simulink model "component_model_with_requirements"  (R2019b)
settings: Solver=VariableStepAuto  StartTime=0.0  StopTime=inf  RelTol=1e-3
settings Model: Creator=anton  LastModifiedBy=scarcia
settings SFSimCC: CustomCodeUndefinedFunction=UseInterfaceOnly

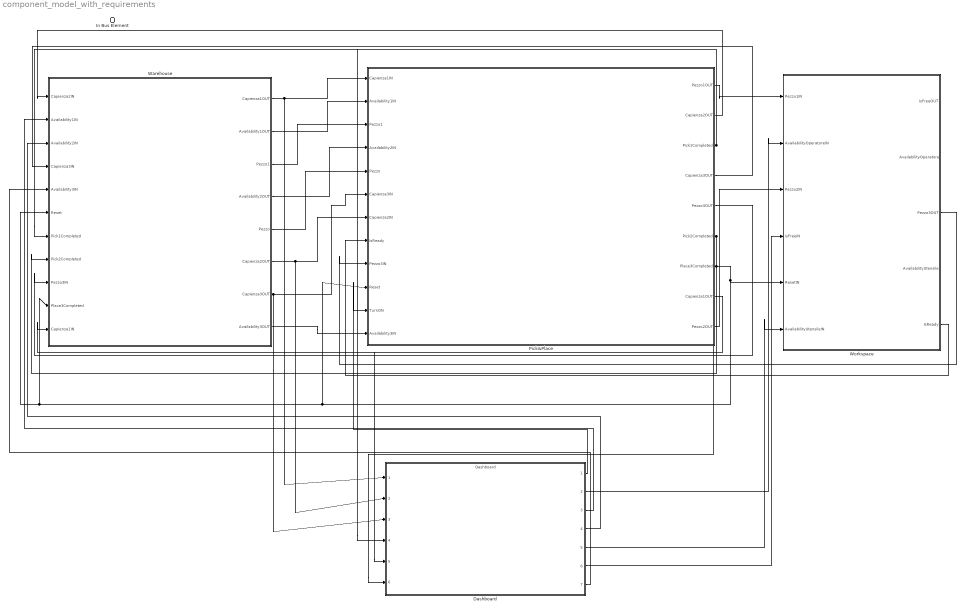
== system component_model_with_requirements ==
  In Bus Element : Inport  PortName=InBus
  Dashboard : ModelReference  ModelNameDialog=Dashboard  SimulationMode=Normal  ModelReferenceVersion=1.7
      settings: PortSchema="{\"entries\":[{\"content\":{\"headerSize\":38,\"margin\":15,\"minimumSpacing\":25,\"sides\":[{\"content\":{\"connectorIds\":[\"In1\",\"In2\",\"In3\",\"In4\",\"In5\",\"In6\"]},\"type\":\"ConnectorPlacement.EquallySpacedRectSide\",\"uuid\":\"84c4e9a6-c7e3-4ff5-8779-8f22ff7ec920\"},{\"content\":{\"connectorIds\":[\"Out1\",\"Out2\",\"Out3\",\"Out4\",\"Out5\",\"Out6\",\"Out7\"],\"side\":\"RIGHT\"},\"type\":\"ConnectorPlacement.EquallySpacedRectSide\",\"uuid\":\"3a8574bf-2f52-453d-9cac-f8720b3c2634\"},{\"content\":{\"connectorIds\":[],\"side\":\"TOP\"},\"type\":\"ConnectorPlacement.EquallySpacedRectSide\",\"uuid\":\"c01d23e2-01e7-488d-9b06-220ab7823b69\"}]},\"type\":\"ConnectorPlacement.EquallySpacedConnector\",\"uuid\":\"4b97af20-a068-43b9-acb3-094aa2dc4c50\"}],\"packageUris\":[\"http:\\/\\/schema.mathworks.com\\/mf0\\/Connector\\/19700101\"],\"version\":\"1.0\"}"
  Pick&Place : Subsystem
      settings: PortSchema="{\"entries\":[{\"content\":{\"headerSize\":26,\"margin\":15,\"minimumSpacing\":25,\"sides\":[{\"content\":{\"connectorIds\":[\"In1\",\"In2\",\"In3\",\"In4\",\"In5\",\"In6\",\"In7\",\"In8\",\"In9\",\"In10\",\"In11\",\"In12\"]},\"type\":\"ConnectorPlacement.EquallySpacedRectSide\",\"uuid\":\"cd5611c0-8a30-4803-bae5-8792d5ed3138\"},{\"content\":{\"connectorIds\":[\"Out1\",\"Out2\",\"Out3\",\"Out4\",\"Out5\",\"Out6\",\"Out7\",\"Out8\",\"Out9\"],\"side\":\"RIGHT\"},\"type\":\"ConnectorPlacement.EquallySpacedRectSide\",\"uuid\":\"19615e04-708c-4dc8-9217-130af3d4c815\"},{\"content\":{\"connectorIds\":[],\"side\":\"TOP\"},\"type\":\"ConnectorPlacement.EquallySpacedRectSide\",\"uuid\":\"bde4fae3-4c2b-4ff8-8efa-5dc73cdd4226\"},{\"content\":{\"connectorIds\":[],\"side\":\"BOTTOM\"},\"type\":\"ConnectorPlacement.EquallySpacedRectSide\",\"uuid\":\"49cfc24f-8487-4a02-9b01-8a859a4a9c32\"}]},\"type\":\"ConnectorPlacement.EquallySpacedConnector\",\"uuid\":\"74f0ebde-c382-4fb1-af99-ecf6372bc12c\"}],\"packageUris\":[\"http:\\/\\/schema.mathworks.com\\/mf0\\/Connector\\/19700101\"],\"version\":\"1.0\"}"
  Warehouse : Subsystem
      settings: PortSchema="{\"entries\":[{\"content\":{\"headerSize\":26,\"margin\":15,\"minimumSpacing\":25,\"sides\":[{\"content\":{\"connectorIds\":[\"In1\",\"In2\",\"In3\",\"In4\",\"In5\",\"In6\",\"In7\",\"In8\",\"In9\",\"In10\",\"In11\"]},\"type\":\"ConnectorPlacement.EquallySpacedRectSide\",\"uuid\":\"cd5611c0-8a30-4803-bae5-8792d5ed3138\"},{\"content\":{\"connectorIds\":[\"Out1\",\"Out2\",\"Out3\",\"Out4\",\"Out5\",\"Out6\",\"Out7\",\"Out8\"],\"side\":\"RIGHT\"},\"type\":\"ConnectorPlacement.EquallySpacedRectSide\",\"uuid\":\"19615e04-708c-4dc8-9217-130af3d4c815\"},{\"content\":{\"connectorIds\":[],\"side\":\"TOP\"},\"type\":\"ConnectorPlacement.EquallySpacedRectSide\",\"uuid\":\"bde4fae3-4c2b-4ff8-8efa-5dc73cdd4226\"}]},\"type\":\"ConnectorPlacement.EquallySpacedConnector\",\"uuid\":\"74f0ebde-c382-4fb1-af99-ecf6372bc12c\"}],\"packageUris\":[\"http:\\/\\/schema.mathworks.com\\/mf0\\/Connector\\/19700101\"],\"version\":\"1.0\"}"
  Workspace : Subsystem
      settings: PortSchema="{\"entries\":[{\"content\":{\"headerSize\":26,\"margin\":15,\"minimumSpacing\":25,\"sides\":[{\"content\":{\"connectorIds\":[\"In1\",\"In2\",\"In3\",\"In4\",\"In5\",\"In6\"]},\"type\":\"ConnectorPlacement.EquallySpacedRectSide\",\"uuid\":\"cd5611c0-8a30-4803-bae5-8792d5ed3138\"},{\"content\":{\"connectorIds\":[\"Out1\",\"Out2\",\"Out3\",\"Out4\",\"Out5\"],\"side\":\"RIGHT\"},\"type\":\"ConnectorPlacement.EquallySpacedRectSide\",\"uuid\":\"19615e04-708c-4dc8-9217-130af3d4c815\"},{\"content\":{\"connectorIds\":[],\"side\":\"TOP\"},\"type\":\"ConnectorPlacement.EquallySpacedRectSide\",\"uuid\":\"bde4fae3-4c2b-4ff8-8efa-5dc73cdd4226\"}]},\"type\":\"ConnectorPlacement.EquallySpacedConnector\",\"uuid\":\"74f0ebde-c382-4fb1-af99-ecf6372bc12c\"}],\"packageUris\":[\"http:\\/\\/schema.mathworks.com\\/mf0\\/Connector\\/19700101\"],\"version\":\"1.0\"}"
  wires:
  Pick&Place/8(Capienza1OUT) -> Warehouse/11(Capienza1IN)
  Pick&Place/2(Capienza2OUT) -> Warehouse/1(Capienza2IN)
  Pick&Place/4(Capienza3OUT) -> Warehouse/4(Capienza3IN)
  Warehouse/1(Capienza1OUT) -> Pick&Place/1(Capienza1IN), Dashboard/1
  Warehouse/6(Capienza2OUT) -> Pick&Place/7(Capienza2IN), Dashboard/2
  Warehouse/3(Pezzo1) -> Pick&Place/3(Pezzo1)
  Warehouse/5(Pezzo) -> Pick&Place/5(Pezzo)
  Warehouse/2(Availability1OUT) -> Pick&Place/2(Availability1IN)
  Warehouse/4(Availability2OUT) -> Pick&Place/4(Availability2IN)
  Warehouse/7(Capienza3OUT) -> Pick&Place/6(Capienza3IN), Dashboard/3
  Pick&Place/1(Pezzo1OUT) -> Workspace/1(Pezzo1IN)
  Pick&Place/9(Pezzo2OUT) -> Workspace/3(Pezzo2IN)
  Workspace/5(IsReady) -> Pick&Place/8(IsReady)
  Workspace/3(Pezzo3OUT) -> Pick&Place/9(Pezzo3IN)
  Pick&Place/5(Pezzo3OUT) -> Warehouse/9(Pezzo3IN)
  Warehouse/8(Availability3OUT) -> Pick&Place/12(Availability3IN)
  Pick&Place/6(Pick2Completed) -> Warehouse/8(Pick2Completed), Dashboard/5
  Pick&Place/3(Pick1Completed) -> Warehouse/7(Pick1Completed), Dashboard/4
  Pick&Place/7(Place3Completed) -> Pick&Place/10(Reset), Warehouse/10(Place3Completed), Warehouse/6(Reset), Workspace/5(ResetIN), Dashboard/6
  Dashboard/3 -> Warehouse/2(Availability1IN)
  Dashboard/4 -> Warehouse/3(Availability2IN)
  Dashboard/2 -> Workspace/2(AvailabilityOperatoreIN)
  Dashboard/5 -> Workspace/6(AvailabilityUtensileIN)
  Dashboard/6 -> Workspace/4(IsFreeIN)
  Dashboard/1 -> Pick&Place/11(TurnON)
  Dashboard/7 -> Warehouse/5(Availability3IN)

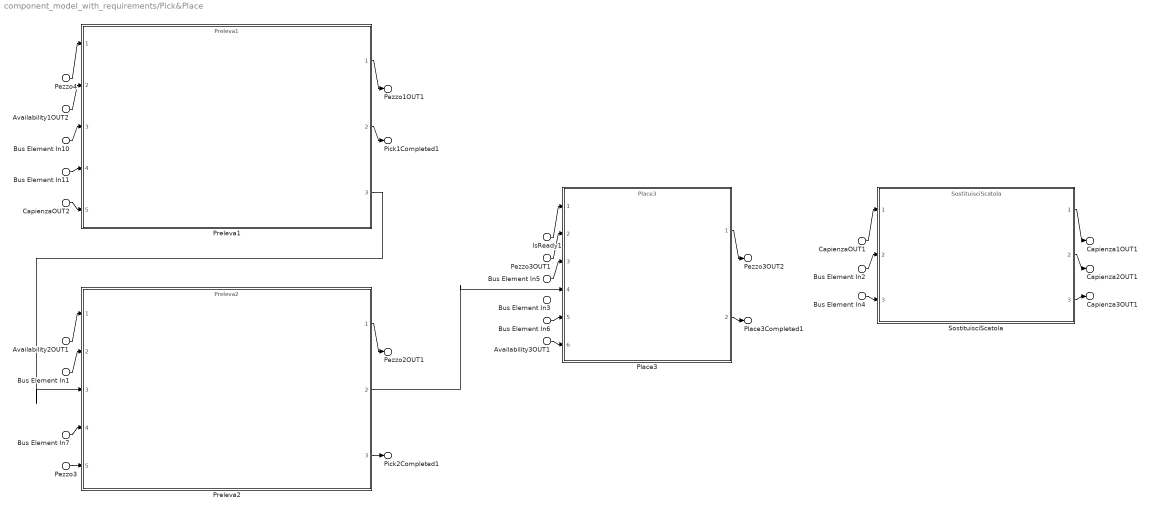
== system component_model_with_requirements/Pick&Place ==
  CapienzaOUT1 : Inport  PortName=Capienza1IN
  CapienzaOUT2 : Inport  PortName=Capienza1IN
  Availability1OUT2 : Inport  Port=2  PortName=Availability1IN
  Pezzo4 : Inport  Port=3  PortName=Pezzo1
  Availability2OUT1 : Inport  Port=4  PortName=Availability2IN
  Pezzo3 : Inport  Port=5  PortName=Pezzo
  Bus Element In4 : Inport  Port=6  PortName=Capienza3IN
  Bus Element In5 : Inport  Port=6  PortName=Capienza3IN
  Bus Element In2 : Inport  Port=7  PortName=Capienza2IN
  Bus Element In1 : Inport  Port=7  PortName=Capienza2IN
  IsReady1 : Inport  Port=8  PortName=IsReady
  Pezzo3OUT1 : Inport  Port=9  PortName=Pezzo3IN
  Bus Element In10 : Inport  Port=10  PortName=Reset
  Bus Element In{3,6..7,11} (4 alike) : Inport  Port=11  PortName=TurnON
  Availability3OUT1 : Inport  Port=12  PortName=Availability3IN
  Place3 : ModelReference  ModelNameDialog=Place3  SimulationMode=Normal  ModelReferenceVersion=1.4
      settings: PortSchema="{\"entries\":[{\"content\":{\"headerSize\":38,\"margin\":15,\"minimumSpacing\":25,\"sides\":[{\"content\":{\"connectorIds\":[\"In1\",\"In2\",\"In3\",\"In4\",\"In5\",\"In6\"]},\"type\":\"ConnectorPlacement.EquallySpacedRectSide\",\"uuid\":\"9a4f82f2-5965-44d2-974e-41fbc79ae372\"},{\"content\":{\"connectorIds\":[\"Out1\",\"Out2\"],\"side\":\"RIGHT\"},\"type\":\"ConnectorPlacement.EquallySpacedRectSide\",\"uuid\":\"61351877-5afa-4df0-ac37-90524965d9bf\"},{\"content\":{\"connectorIds\":[],\"side\":\"TOP\"},\"type\":\"ConnectorPlacement.EquallySpacedRectSide\",\"uuid\":\"d32a260f-cbbe-4f7d-b4af-6968319b36d3\"}]},\"type\":\"ConnectorPlacement.EquallySpacedConnector\",\"uuid\":\"7cd8970c-ddce-45f4-acf5-ff169a620ce7\"}],\"packageUris\":[\"http:\\/\\/schema.mathworks.com\\/mf0\\/Connector\\/19700101\"],\"version\":\"1.0\"}"
  Preleva1 : ModelReference  ModelNameDialog=Preleva1  SimulationMode=Normal  ModelReferenceVersion=1.4
      settings: PortSchema="{\"entries\":[{\"content\":{\"headerSize\":38,\"margin\":15,\"minimumSpacing\":25,\"sides\":[{\"content\":{\"connectorIds\":[\"In1\",\"In2\",\"In3\",\"In4\",\"In5\"]},\"type\":\"ConnectorPlacement.EquallySpacedRectSide\",\"uuid\":\"9a4f82f2-5965-44d2-974e-41fbc79ae372\"},{\"content\":{\"connectorIds\":[\"Out1\",\"Out2\",\"Out3\"],\"side\":\"RIGHT\"},\"type\":\"ConnectorPlacement.EquallySpacedRectSide\",\"uuid\":\"61351877-5afa-4df0-ac37-90524965d9bf\"},{\"content\":{\"connectorIds\":[],\"side\":\"TOP\"},\"type\":\"ConnectorPlacement.EquallySpacedRectSide\",\"uuid\":\"d32a260f-cbbe-4f7d-b4af-6968319b36d3\"}]},\"type\":\"ConnectorPlacement.EquallySpacedConnector\",\"uuid\":\"7cd8970c-ddce-45f4-acf5-ff169a620ce7\"}],\"packageUris\":[\"http:\\/\\/schema.mathworks.com\\/mf0\\/Connector\\/19700101\"],\"version\":\"1.0\"}"
  Preleva2 : ModelReference  ModelNameDialog=Preleva2  SimulationMode=Normal  ModelReferenceVersion=1.4
      settings: PortSchema="{\"entries\":[{\"content\":{\"headerSize\":38,\"margin\":15,\"minimumSpacing\":25,\"sides\":[{\"content\":{\"connectorIds\":[\"In1\",\"In2\",\"In3\",\"In4\",\"In5\"]},\"type\":\"ConnectorPlacement.EquallySpacedRectSide\",\"uuid\":\"9a4f82f2-5965-44d2-974e-41fbc79ae372\"},{\"content\":{\"connectorIds\":[\"Out1\",\"Out2\",\"Out3\"],\"side\":\"RIGHT\"},\"type\":\"ConnectorPlacement.EquallySpacedRectSide\",\"uuid\":\"61351877-5afa-4df0-ac37-90524965d9bf\"},{\"content\":{\"connectorIds\":[],\"side\":\"TOP\"},\"type\":\"ConnectorPlacement.EquallySpacedRectSide\",\"uuid\":\"d32a260f-cbbe-4f7d-b4af-6968319b36d3\"}]},\"type\":\"ConnectorPlacement.EquallySpacedConnector\",\"uuid\":\"7cd8970c-ddce-45f4-acf5-ff169a620ce7\"}],\"packageUris\":[\"http:\\/\\/schema.mathworks.com\\/mf0\\/Connector\\/19700101\"],\"version\":\"1.0\"}"
  SostituisciScatola : ModelReference  ModelNameDialog=SostituisciScatola  SimulationMode=Normal  ModelReferenceVersion=1.4
      settings: PortSchema="{\"entries\":[{\"content\":{\"headerSize\":38,\"margin\":15,\"minimumSpacing\":25,\"sides\":[{\"content\":{\"connectorIds\":[\"In1\",\"In2\",\"In3\"]},\"type\":\"ConnectorPlacement.EquallySpacedRectSide\",\"uuid\":\"3b3968ce-44ce-4ff1-b340-b6df1f6f3847\"},{\"content\":{\"connectorIds\":[\"Out1\",\"Out2\",\"Out3\"],\"side\":\"RIGHT\"},\"type\":\"ConnectorPlacement.EquallySpacedRectSide\",\"uuid\":\"732ea1f5-375c-4ad6-872e-d3b4542e6ff4\"},{\"content\":{\"connectorIds\":[],\"side\":\"TOP\"},\"type\":\"ConnectorPlacement.EquallySpacedRectSide\",\"uuid\":\"c54c1e69-891a-4a92-a343-95705edc23ec\"}]},\"type\":\"ConnectorPlacement.EquallySpacedConnector\",\"uuid\":\"4605bdf0-2cd0-40bf-899c-a64563e2f0be\"}],\"packageUris\":[\"http:\\/\\/schema.mathworks.com\\/mf0\\/Connector\\/19700101\"],\"version\":\"1.0\"}"
  Pezzo1OUT1 : Outport  VectorParamsAs1DForOutWhenUnconnected=off  PortName=Pezzo1OUT
  Capienza2OUT1 : Outport  Port=2  VectorParamsAs1DForOutWhenUnconnected=off  PortName=Capienza2OUT
  Pick1Completed1 : Outport  Port=3  VectorParamsAs1DForOutWhenUnconnected=off  PortName=Pick1Completed
  Capienza3OUT1 : Outport  Port=4  VectorParamsAs1DForOutWhenUnconnected=off  PortName=Capienza3OUT
  Pezzo3OUT2 : Outport  Port=5  VectorParamsAs1DForOutWhenUnconnected=off  PortName=Pezzo3OUT
  Pick2Completed1 : Outport  Port=6  VectorParamsAs1DForOutWhenUnconnected=off  PortName=Pick2Completed
  Place3Completed1 : Outport  Port=7  VectorParamsAs1DForOutWhenUnconnected=off  PortName=Place3Completed
  Capienza1OUT1 : Outport  Port=8  VectorParamsAs1DForOutWhenUnconnected=off  PortName=Capienza1OUT
  Pezzo2OUT1 : Outport  Port=9  VectorParamsAs1DForOutWhenUnconnected=off  PortName=Pezzo2OUT
  wires:
  Availability1OUT2/1 -> Preleva1/2
  Pezzo4/1 -> Preleva1/1
  Bus Element In10/1 -> Preleva1/3
  Bus Element In11/1 -> Preleva1/4
  CapienzaOUT2/1 -> Preleva1/5
  Preleva1/1 -> Pezzo1OUT1/1
  Preleva1/2 -> Pick1Completed1/1
  Availability2OUT1/1 -> Preleva2/1
  Bus Element In1/1 -> Preleva2/2
  Preleva1/3 -> Preleva2/3
  Bus Element In7/1 -> Preleva2/4
  Pezzo3/1 -> Preleva2/5
  Preleva2/1 -> Pezzo2OUT1/1
  Preleva2/3 -> Pick2Completed1/1
  Availability3OUT1/1 -> Place3/6
  IsReady1/1 -> Place3/1
  Pezzo3OUT1/1 -> Place3/2
  Bus Element In5/1 -> Place3/3
  Preleva2/2 -> Place3/4
  Bus Element In6/1 -> Place3/5
  Place3/1 -> Pezzo3OUT2/1
  Place3/2 -> Place3Completed1/1
  CapienzaOUT1/1 -> SostituisciScatola/1
  Bus Element In2/1 -> SostituisciScatola/2
  Bus Element In4/1 -> SostituisciScatola/3
  SostituisciScatola/1 -> Capienza1OUT1/1
  SostituisciScatola/2 -> Capienza2OUT1/1
  SostituisciScatola/3 -> Capienza3OUT1/1

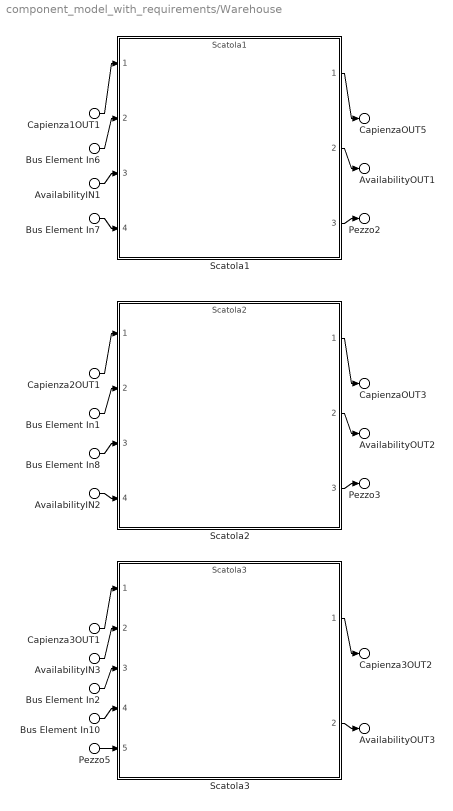
== system component_model_with_requirements/Warehouse ==
  Capienza2OUT1 : Inport  PortName=Capienza2IN
  AvailabilityIN1 : Inport  Port=2  PortName=Availability1IN
  AvailabilityIN2 : Inport  Port=3  PortName=Availability2IN
  Capienza3OUT1 : Inport  Port=4  PortName=Capienza3IN
  AvailabilityIN3 : Inport  Port=5  PortName=Availability3IN
  Bus Element In6 : Inport  Port=6  PortName=Reset
  Bus Element In1 : Inport  Port=6  PortName=Reset
  Bus Element In7 : Inport  Port=7  PortName=Pick1Completed
  Bus Element In2 : Inport  Port=7  PortName=Pick1Completed
  Bus Element In8 : Inport  Port=8  PortName=Pick2Completed
  Pezzo5 : Inport  Port=9  PortName=Pezzo3IN
  Bus Element In10 : Inport  Port=10  PortName=Place3Completed
  Capienza1OUT1 : Inport  Port=11  PortName=Capienza1IN
  Scatola1 : ModelReference  ModelNameDialog=Scatola1  SimulationMode=Normal  ModelReferenceVersion=1.4
      settings: PortSchema="{\"entries\":[{\"content\":{\"headerSize\":38,\"margin\":15,\"minimumSpacing\":25,\"sides\":[{\"content\":{\"connectorIds\":[\"In1\",\"In2\",\"In3\",\"In4\"]},\"type\":\"ConnectorPlacement.EquallySpacedRectSide\",\"uuid\":\"8ca3f795-bcf3-41f9-ab0e-0c7be44eb4b6\"},{\"content\":{\"connectorIds\":[\"Out1\",\"Out2\",\"Out3\"],\"side\":\"RIGHT\"},\"type\":\"ConnectorPlacement.EquallySpacedRectSide\",\"uuid\":\"3b3dc70a-b452-493d-8b71-47a0b7c01cc2\"},{\"content\":{\"connectorIds\":[],\"side\":\"TOP\"},\"type\":\"ConnectorPlacement.EquallySpacedRectSide\",\"uuid\":\"cab02728-e64d-4893-9add-95830667e0b5\"}]},\"type\":\"ConnectorPlacement.EquallySpacedConnector\",\"uuid\":\"f743a47e-71b4-48a2-b6e9-fcbf02047a86\"}],\"packageUris\":[\"http:\\/\\/schema.mathworks.com\\/mf0\\/Connector\\/19700101\"],\"version\":\"1.0\"}"
  Scatola2 : ModelReference  ModelNameDialog=Scatola2  SimulationMode=Normal  ModelReferenceVersion=1.3
      settings: PortSchema="{\"entries\":[{\"content\":{\"headerSize\":38,\"margin\":15,\"minimumSpacing\":25,\"sides\":[{\"content\":{\"connectorIds\":[\"In1\",\"In2\",\"In3\",\"In4\"]},\"type\":\"ConnectorPlacement.EquallySpacedRectSide\",\"uuid\":\"cd5611c0-8a30-4803-bae5-8792d5ed3138\"},{\"content\":{\"connectorIds\":[\"Out1\",\"Out2\",\"Out3\"],\"side\":\"RIGHT\"},\"type\":\"ConnectorPlacement.EquallySpacedRectSide\",\"uuid\":\"19615e04-708c-4dc8-9217-130af3d4c815\"},{\"content\":{\"connectorIds\":[],\"side\":\"TOP\"},\"type\":\"ConnectorPlacement.EquallySpacedRectSide\",\"uuid\":\"bde4fae3-4c2b-4ff8-8efa-5dc73cdd4226\"}]},\"type\":\"ConnectorPlacement.EquallySpacedConnector\",\"uuid\":\"74f0ebde-c382-4fb1-af99-ecf6372bc12c\"}],\"packageUris\":[\"http:\\/\\/schema.mathworks.com\\/mf0\\/Connector\\/19700101\"],\"version\":\"1.0\"}"
  Scatola3 : ModelReference  ModelNameDialog=Scatola3  SimulationMode=Normal  ModelReferenceVersion=1.3
      settings: PortSchema="{\"entries\":[{\"content\":{\"headerSize\":38,\"margin\":15,\"minimumSpacing\":25,\"sides\":[{\"content\":{\"connectorIds\":[\"In1\",\"In2\",\"In3\",\"In4\",\"In5\"]},\"type\":\"ConnectorPlacement.EquallySpacedRectSide\",\"uuid\":\"cd5611c0-8a30-4803-bae5-8792d5ed3138\"},{\"content\":{\"connectorIds\":[\"Out1\",\"Out2\"],\"side\":\"RIGHT\"},\"type\":\"ConnectorPlacement.EquallySpacedRectSide\",\"uuid\":\"19615e04-708c-4dc8-9217-130af3d4c815\"},{\"content\":{\"connectorIds\":[],\"side\":\"TOP\"},\"type\":\"ConnectorPlacement.EquallySpacedRectSide\",\"uuid\":\"bde4fae3-4c2b-4ff8-8efa-5dc73cdd4226\"}]},\"type\":\"ConnectorPlacement.EquallySpacedConnector\",\"uuid\":\"74f0ebde-c382-4fb1-af99-ecf6372bc12c\"}],\"packageUris\":[\"http:\\/\\/schema.mathworks.com\\/mf0\\/Connector\\/19700101\"],\"version\":\"1.0\"}"
  CapienzaOUT5 : Outport  VectorParamsAs1DForOutWhenUnconnected=off  PortName=Capienza1OUT
  AvailabilityOUT1 : Outport  Port=2  VectorParamsAs1DForOutWhenUnconnected=off  PortName=Availability1OUT
  Pezzo2 : Outport  Port=3  VectorParamsAs1DForOutWhenUnconnected=off  PortName=Pezzo1
  AvailabilityOUT2 : Outport  Port=4  VectorParamsAs1DForOutWhenUnconnected=off  PortName=Availability2OUT
  Pezzo3 : Outport  Port=5  VectorParamsAs1DForOutWhenUnconnected=off  PortName=Pezzo
  CapienzaOUT3 : Outport  Port=6  VectorParamsAs1DForOutWhenUnconnected=off  PortName=Capienza2OUT
  Capienza3OUT2 : Outport  Port=7  VectorParamsAs1DForOutWhenUnconnected=off  PortName=Capienza3OUT
  AvailabilityOUT3 : Outport  Port=8  VectorParamsAs1DForOutWhenUnconnected=off  PortName=Availability3OUT
  wires:
  AvailabilityIN1/1 -> Scatola1/3
  Capienza1OUT1/1 -> Scatola1/1
  Bus Element In7/1 -> Scatola1/4
  Bus Element In6/1 -> Scatola1/2
  Scatola1/1 -> CapienzaOUT5/1
  Scatola1/2 -> AvailabilityOUT1/1
  Scatola1/3 -> Pezzo2/1
  AvailabilityIN2/1 -> Scatola2/4
  Capienza2OUT1/1 -> Scatola2/1
  Bus Element In8/1 -> Scatola2/3
  Bus Element In1/1 -> Scatola2/2
  Scatola2/1 -> CapienzaOUT3/1
  Scatola2/2 -> AvailabilityOUT2/1
  Scatola2/3 -> Pezzo3/1
  AvailabilityIN3/1 -> Scatola3/2
  Capienza3OUT1/1 -> Scatola3/1
  Pezzo5/1 -> Scatola3/5
  Bus Element In10/1 -> Scatola3/4
  Scatola3/1 -> Capienza3OUT2/1
  Scatola3/2 -> AvailabilityOUT3/1
  Bus Element In2/1 -> Scatola3/3

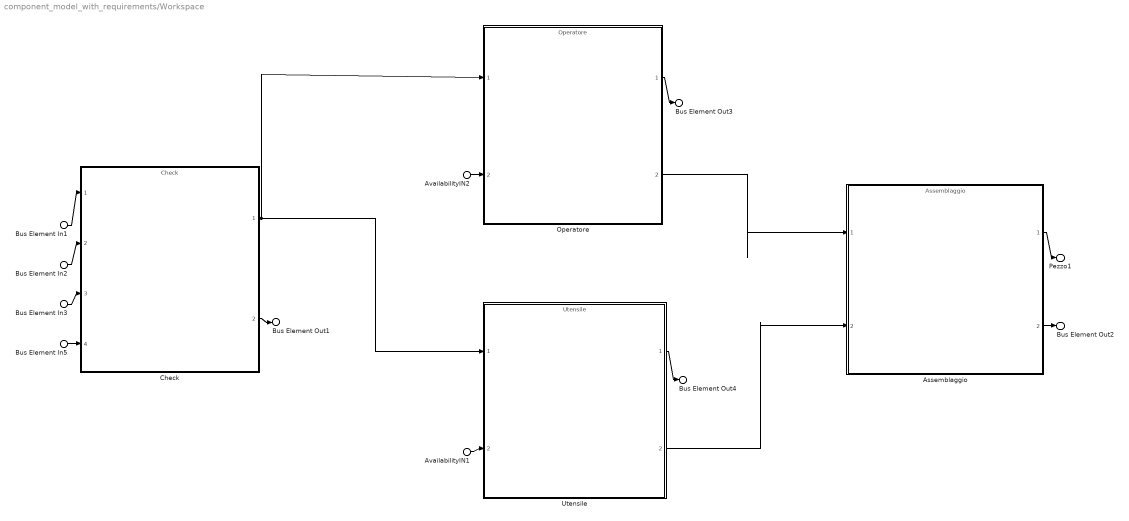
== system component_model_with_requirements/Workspace ==
  Bus Element In1 : Inport  PortName=Pezzo1IN
  AvailabilityIN2 : Inport  Port=2  PortName=AvailabilityOperatoreIN
  Bus Element In2 : Inport  Port=3  PortName=Pezzo2IN
  Bus Element In3 : Inport  Port=4  PortName=IsFreeIN
  Bus Element In5 : Inport  Port=5  PortName=ResetIN
  AvailabilityIN1 : Inport  Port=6  PortName=AvailabilityUtensileIN
  Assemblaggio : ModelReference  ModelNameDialog=Assemblaggio  SimulationMode=Normal  ModelReferenceVersion=1.2
      settings: PortSchema="{\"entries\":[{\"content\":{\"headerSize\":38,\"margin\":15,\"minimumSpacing\":25,\"sides\":[{\"content\":{\"connectorIds\":[\"In1\",\"In2\"]},\"type\":\"ConnectorPlacement.EquallySpacedRectSide\",\"uuid\":\"cd5611c0-8a30-4803-bae5-8792d5ed3138\"},{\"content\":{\"connectorIds\":[\"Out1\",\"Out2\"],\"side\":\"RIGHT\"},\"type\":\"ConnectorPlacement.EquallySpacedRectSide\",\"uuid\":\"19615e04-708c-4dc8-9217-130af3d4c815\"},{\"content\":{\"connectorIds\":[],\"side\":\"TOP\"},\"type\":\"ConnectorPlacement.EquallySpacedRectSide\",\"uuid\":\"bde4fae3-4c2b-4ff8-8efa-5dc73cdd4226\"}]},\"type\":\"ConnectorPlacement.EquallySpacedConnector\",\"uuid\":\"74f0ebde-c382-4fb1-af99-ecf6372bc12c\"}],\"packageUris\":[\"http:\\/\\/schema.mathworks.com\\/mf0\\/Connector\\/19700101\"],\"version\":\"1.0\"}"
  Check : ModelReference  ModelNameDialog=Check  SimulationMode=Normal  ModelReferenceVersion=1.3
      settings: PortSchema="{\"entries\":[{\"content\":{\"headerSize\":38,\"margin\":15,\"minimumSpacing\":25,\"sides\":[{\"content\":{\"connectorIds\":[\"In1\",\"In2\",\"In3\",\"In4\"]},\"type\":\"ConnectorPlacement.EquallySpacedRectSide\",\"uuid\":\"cd5611c0-8a30-4803-bae5-8792d5ed3138\"},{\"content\":{\"connectorIds\":[\"Out1\",\"Out2\"],\"side\":\"RIGHT\"},\"type\":\"ConnectorPlacement.EquallySpacedRectSide\",\"uuid\":\"19615e04-708c-4dc8-9217-130af3d4c815\"},{\"content\":{\"connectorIds\":[],\"side\":\"TOP\"},\"type\":\"ConnectorPlacement.EquallySpacedRectSide\",\"uuid\":\"bde4fae3-4c2b-4ff8-8efa-5dc73cdd4226\"}]},\"type\":\"ConnectorPlacement.EquallySpacedConnector\",\"uuid\":\"74f0ebde-c382-4fb1-af99-ecf6372bc12c\"}],\"packageUris\":[\"http:\\/\\/schema.mathworks.com\\/mf0\\/Connector\\/19700101\"],\"version\":\"1.0\"}"
  Operatore : ModelReference  ModelNameDialog=Operatore  SimulationMode=Normal  ModelReferenceVersion=1.2
      settings: PortSchema="{\"entries\":[{\"content\":{\"headerSize\":38,\"margin\":15,\"minimumSpacing\":25,\"sides\":[{\"content\":{\"connectorIds\":[\"In1\",\"In2\"]},\"type\":\"ConnectorPlacement.EquallySpacedRectSide\",\"uuid\":\"cd5611c0-8a30-4803-bae5-8792d5ed3138\"},{\"content\":{\"connectorIds\":[\"Out1\",\"Out2\"],\"side\":\"RIGHT\"},\"type\":\"ConnectorPlacement.EquallySpacedRectSide\",\"uuid\":\"19615e04-708c-4dc8-9217-130af3d4c815\"},{\"content\":{\"connectorIds\":[],\"side\":\"TOP\"},\"type\":\"ConnectorPlacement.EquallySpacedRectSide\",\"uuid\":\"bde4fae3-4c2b-4ff8-8efa-5dc73cdd4226\"}]},\"type\":\"ConnectorPlacement.EquallySpacedConnector\",\"uuid\":\"74f0ebde-c382-4fb1-af99-ecf6372bc12c\"}],\"packageUris\":[\"http:\\/\\/schema.mathworks.com\\/mf0\\/Connector\\/19700101\"],\"version\":\"1.0\"}"
  Utensile : ModelReference  ModelNameDialog=Utensile  SimulationMode=Normal  ModelReferenceVersion=1.2
      settings: PortSchema="{\"entries\":[{\"content\":{\"headerSize\":38,\"margin\":15,\"minimumSpacing\":25,\"sides\":[{\"content\":{\"connectorIds\":[\"In1\",\"In2\"]},\"type\":\"ConnectorPlacement.EquallySpacedRectSide\",\"uuid\":\"cd5611c0-8a30-4803-bae5-8792d5ed3138\"},{\"content\":{\"connectorIds\":[\"Out1\",\"Out2\"],\"side\":\"RIGHT\"},\"type\":\"ConnectorPlacement.EquallySpacedRectSide\",\"uuid\":\"19615e04-708c-4dc8-9217-130af3d4c815\"},{\"content\":{\"connectorIds\":[],\"side\":\"TOP\"},\"type\":\"ConnectorPlacement.EquallySpacedRectSide\",\"uuid\":\"bde4fae3-4c2b-4ff8-8efa-5dc73cdd4226\"}]},\"type\":\"ConnectorPlacement.EquallySpacedConnector\",\"uuid\":\"74f0ebde-c382-4fb1-af99-ecf6372bc12c\"}],\"packageUris\":[\"http:\\/\\/schema.mathworks.com\\/mf0\\/Connector\\/19700101\"],\"version\":\"1.0\"}"
  Bus Element Out1 : Outport  VectorParamsAs1DForOutWhenUnconnected=off  PortName=IsFreeOUT
  Bus Element Out3 : Outport  Port=2  VectorParamsAs1DForOutWhenUnconnected=off  PortName=AvailabilityOperatore
  Pezzo1 : Outport  Port=3  VectorParamsAs1DForOutWhenUnconnected=off  PortName=Pezzo3OUT
  Bus Element Out4 : Outport  Port=4  VectorParamsAs1DForOutWhenUnconnected=off  PortName=AvailabilityUtensile
  Bus Element Out2 : Outport  Port=5  VectorParamsAs1DForOutWhenUnconnected=off  PortName=IsReady
  wires:
  Bus Element In3/1 -> Check/3
  Bus Element In1/1 -> Check/1
  Bus Element In2/1 -> Check/2
  Bus Element In5/1 -> Check/4
  Check/2 -> Bus Element Out1/1
  Check/1 -> Operatore/1, Utensile/1
  AvailabilityIN2/1 -> Operatore/2
  Operatore/1 -> Bus Element Out3/1
  AvailabilityIN1/1 -> Utensile/2
  Utensile/1 -> Bus Element Out4/1
  Operatore/2 -> Assemblaggio/1
  Utensile/2 -> Assemblaggio/2
  Assemblaggio/2 -> Bus Element Out2/1
  Assemblaggio/1 -> Pezzo1/1
